simulink model "VSI_Space_Vector_PWM"  (R2020b)
settings: Solver=ode45  StartTime=0.0  StopTime=5/fc  MaxStep=1e-5  RelTol=1e-3  EnableMultiTasking=on
InitFcn:
  | Vdc=400;
  | Ts=2e-6; %Simulation sampling time
  | fc = 50;
  | fs = 10000;
  | shift = 0;
  | m = 1;
StopFcn:
  | clc
  | figure(1);
  | plot(a(:,1),a(:,2),'-b',b(:,1),b(:,2),'-r');
  | axis equal;
  | grid;
  | title('Space Vector PWM');
  | 
model workspace (MAT data in the model file):
  Param = Simulink.Parameter
  Param.Value = 25
  Param.DataType = 'auto'
  Param.Dimensions = [1 1]
  sw_array = reshape([0 0 0 1 0 0 1 1 0 1 1 1 1 1 0 1 0 0 0 0 0 0 0 0 0 1 0 1 1 0 1 1 1 1 1 0 0 1 0 0 0 0 0 0 0 0 1 0 0 1 1 1 1 1 0 1 1 0 1 0 0 0 0 0 0 0 0 0 1 0 1 1 1 1 1 0 1 1 0 0 1 0 0 0 0 0 0 0 0 1 1 0 1 1 1 1 1 0 1 0 0 1 0 0 0 0 0 0 1 0 0 1 0 1 1 1 1 1 0 1 1 0 0 0 0 0], [3 7 6])
libraries: powerlib x20, simulink x2
settings Model: Creator=sample  LastModifiedBy=Karim
settings DataIOCC: LimitDataPoints=on  SaveFormat=Array  SignalLoggingSaveFormat=ModelDataLogs  ReturnWorkspaceOutputs=off
settings OptimizationCC: ExpressionDepthLimit=2147483647  LifeSpan=inf
settings DebuggingCC: UnderspecifiedInitializationDetection=Classic  MergeDetectMultiDrivingBlocksExec=none  SolverPrmCheckMsg=warning  FcnCallInpInsideContextMsg=warning  StateNameClashWarn=warning  SFUnexpectedBacktrackingDiag=warning  SFNoUnconditionalDefaultTransitionDiag=warning  SFExecutionAtInitializationDiag=none  ArithmeticOperatorsInVariantConditions=warning
settings HardwareCC: ProdBitPerPointer=32  ProdBitPerSizeT=32  ProdBitPerPtrDiffT=32  ProdLargestAtomicFloat=None  ProdIntDivRoundTo=Undefined  ProdEndianess=Unspecified  ProdWordSize=32  ProdHWDeviceType=32-bit Generic
settings ModelReferenceCC: PropagateSignalLabelsOutOfModel=off
settings SFSimCC: SimUseLocalCustomCode=off  CustomCodeUndefinedFunction=UseInterfaceOnly
settings RTWCC: RTWUseLocalCustomCode=off
settings CodeAppCC: StateflowObjectComments=on
settings GRTTargetCC: TargetLangStandard=C89/C90 (ANSI)  CombineOutputUpdateFcns=off  GRTInterface=on
settings ConfigComp: CovMetricSettings=dw  CovSaveCumulativeToWorkspaceVar=on  CovSaveSingleToWorkspaceVar=on  CovExternalEMLEnable=off
settings SimscapeCC: SimscapeNormalizeSystem=off

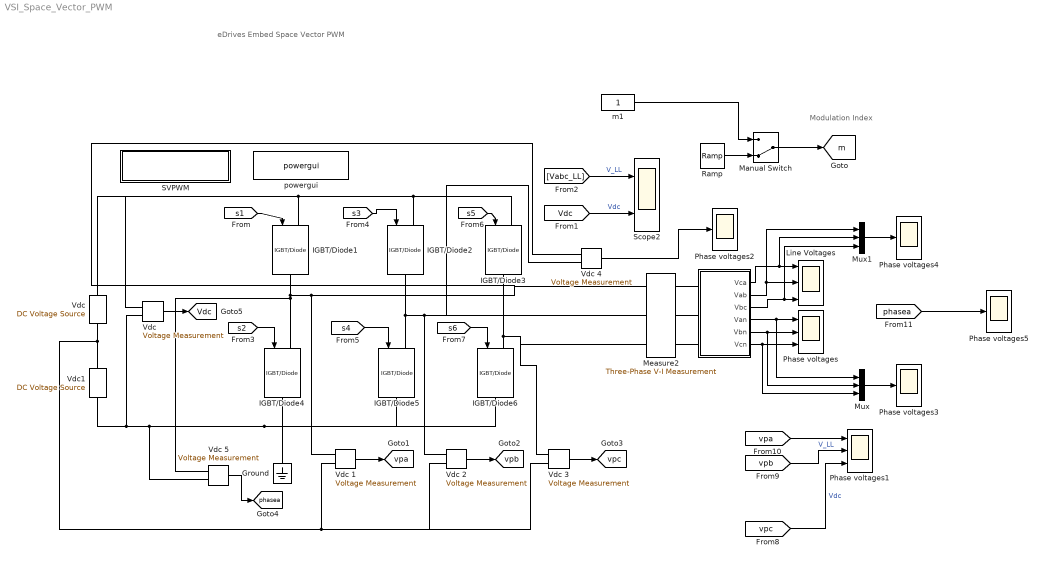
== system VSI_Space_Vector_PWM ==
  note: Modulation Index
  note: eDrives Embed
      |
      |   Space Vector  PWM
  " " : Subsystem
  Ground : powerlib/Elements/Ground  LConnTagsString=a
  IGBT/Diode{1..6} (6 alike) : powerlib/Power Electronics/IGBT//Diode  Ron=1e-3  Rs=1e5  Cs=inf  Measurements=off
  Line Voltages : Scope  NumInputPorts=3
  Manual Switch : ManualSwitch  CurrentSetting=0
  Measure2 : powerlib/Measurements/Three-Phase V-I Measurement  VoltageMeasurement=phase-to-phase  SetLabelV=on  LabelV=Vabc_LL  Vpu=off  VpuLL=off  CurrentMeasurement=no  SetLabelI=off  LabelI=I1  Ipu=off  Pbase=1e3  Vbase=380  OutputType=Magnitude  PhasorSimulation=off  PSBequivalent=0
  Mux : Mux  Inputs=3
  Mux1 : Mux  Inputs=3
  Phase voltages : Scope  NumInputPorts=3
  Phase voltages1 : Scope  NumInputPorts=3
  Phase voltages{2..5} (4 alike) : Scope
  Ramp : simulink/Sources/Ramp  slope=5  start=0  InitialOutput=0.5
  SVPWM : Subsystem
  Scope2 : Scope  NumInputPorts=2
  Vdc : powerlib/Electrical Sources/DC Voltage Source  Amplitude=200  Measurements=None
  Vdc {,1..5} (6 alike) : powerlib/Measurements/Voltage Measurement  Tag=PoWeRsYsTeMmEaSuReMeNt  PhasorSimulation=off  OutputType=Magnitude  PSBequivalent=0
  Vdc1 : powerlib/Electrical Sources/DC Voltage Source  Amplitude=200  Measurements=None
  m1 : Constant  SampleTime=Ts
  powergui : powerlib/powergui  Priority=1  SimulationMode=Discrete  SampleTime=1e-6  frequency=60  Iterations=50  frequencyindice=0  Pbase=100e6  ErrMax=1e-4  UnitsV=kV  UnitsW=MW  buscounter=0  FunctionMessages=off  echomessages=off  EnableUseOfTLC=off  CurrentSourceSwitches=off  DisableSnubberDevices=off  DisableRonSwitches=off  DisableVfSwitches=off  DisplayEquations=off  AutomaticDiscreteSolvers=off  SolverType=Tustin  Interpol=off  ExternalGateDelay=off  methode=off  Ts=0  x0status=blocks  SPID=on  SwTol=0  HookPort=off  NonlinearTolerance=1e-4  nMaxIteration=100  ContinueOnMaxIteration=off  RestoreLinks=warning  ResistiveCurrentMeasurement=off  Frange=[0:2:500]  Ylog=off  Xlog=on  ShowGrid=off  save=off  variable=ZData  structure=sv2  ZoomFFT=off  StartTime=0  cycles=2  DisplayStyle=1  fundamental=50  FreqAxis=on  MaxFrequency=650  frequencyindicesteady=1  RmsSteady=1  display=off
  tag scope: Vdc=global, m=global, phasea=global, vpa=global, vpb=global, vpc=global
  wires:
  "Vdc "/1 -> [Vdc]
  " "/4(Van) -> Mux/1, Phase voltages/1
  " "/5(Vbn) -> Mux/2, Phase voltages/2
  " "/6(Vcn) -> Mux/3, Phase voltages/3
  [Vabc_LL] -> Scope2/1  "V_LL"
  [Vdc] -> Scope2/2  "Vdc"
  [s1] -> IGBT/Diode1/1
  [s2] -> IGBT/Diode4/1
  [s3] -> IGBT/Diode2/1
  [s4] -> IGBT/Diode5/1
  [s5] -> IGBT/Diode3/1
  [s6] -> IGBT/Diode6/1
  " "/1(Vca) -> Mux1/2, Line Voltages/1
  " "/2(Vab) -> Mux1/1, Line Voltages/2
  " "/3(Vbc) -> Line Voltages/3, Mux1/3
  m1/1 -> Manual Switch/1
  Manual Switch/1 -> [m]
  Ramp/1 -> Manual Switch/2
  Vdc 1/1 -> [vpa]
  Vdc 2/1 -> [vpb]
  Vdc 3/1 -> [vpc]
  [vpb] -> Phase voltages1/2  "V_LL"
  [vpc] -> Phase voltages1/3  "Vdc"
  [vpa] -> Phase voltages1/1
  Vdc 4/1 -> Phase voltages2/1
  Mux/1 -> Phase voltages3/1
  Mux1/1 -> Phase voltages4/1
  Vdc 5/1 -> [phasea]
  [phasea] -> Phase voltages5/1
  connections:
  Measure2/RConn1 -- " "/LConn1
  Measure2/RConn2 -- " "/LConn2
  " "/LConn3 -- Measure2/RConn3
  IGBT/Diode2/LConn1 -- IGBT/Diode3/LConn1 -- Vdc/RConn1 -- "Vdc "/LConn1 -- IGBT/Diode1/LConn1
  IGBT/Diode1/RConn1 -- Measure2/LConn1 -- Vdc 4/LConn1 -- Vdc 1/LConn1 -- IGBT/Diode4/LConn1 -- Vdc 5/LConn1
  IGBT/Diode5/RConn1 -- IGBT/Diode6/RConn1 -- Ground/LConn1 -- IGBT/Diode4/RConn1 -- Vdc 5/LConn2 -- Vdc1/LConn1 -- "Vdc "/LConn2
  IGBT/Diode3/RConn1 -- Measure2/LConn3 -- Vdc 3/LConn1 -- IGBT/Diode6/LConn1
  IGBT/Diode5/LConn1 -- Measure2/LConn2 -- Vdc 4/LConn2 -- Vdc 2/LConn1 -- IGBT/Diode2/RConn1
  Vdc 1/LConn2 -- Vdc/LConn1 -- Vdc1/RConn1 -- Vdc 3/LConn2 -- Vdc 2/LConn2

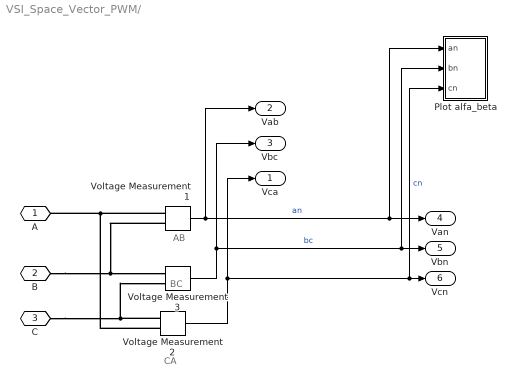
== system VSI_Space_Vector_PWM/  ==
  note: CA
  note: BC
  note: AB
  Plot alfa_beta : Subsystem
  Voltage Measurement1 : powerlib/Measurements/Voltage Measurement  PhasorSimulation=off  OutputType=Complex  PSBequivalent=0
  Voltage Measurement2 : powerlib/Measurements/Voltage Measurement  PhasorSimulation=off  OutputType=Complex  PSBequivalent=0
  Voltage Measurement3 : powerlib/Measurements/Voltage Measurement  PhasorSimulation=off  OutputType=Complex  PSBequivalent=0
  A : PMIOPort  Side=Left
  B : PMIOPort  Port=2  Side=Left
  C : PMIOPort  Port=3  Side=Left
  Vca : Outport
  Vab : Outport  Port=2
  Vbc : Outport  Port=3
  Van : Outport  Port=4
  Vbn : Outport  Port=5
  Vcn : Outport  Port=6
  wires:
  Voltage Measurement3/1 -> Plot alfa_beta/2(bn), Vbn/1, Vbc/1  "bc"
  Voltage Measurement1/1 -> Plot alfa_beta/1(an), Van/1, Vab/1  "an"
  Voltage Measurement2/1 -> Plot alfa_beta/3(cn), Vcn/1, Vca/1  "cn"
  connections:
  Voltage Measurement1/LConn2 -- B/RConn1 -- Voltage Measurement3/LConn1
  Voltage Measurement2/LConn1 -- C/RConn1 -- Voltage Measurement3/LConn2
  Voltage Measurement1/LConn1 -- Voltage Measurement2/LConn2 -- A/RConn1

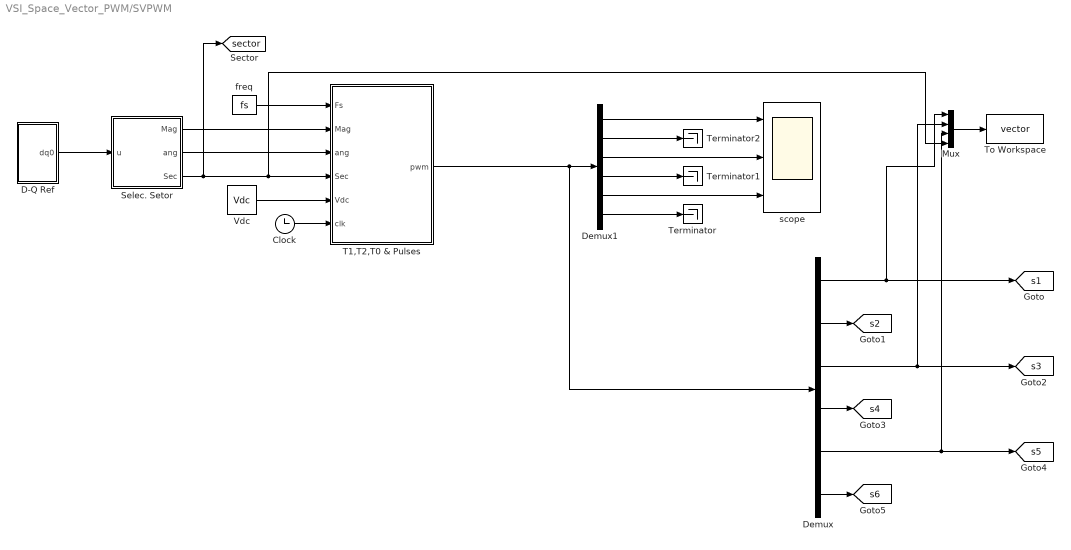
== system VSI_Space_Vector_PWM/SVPWM ==
  " T1,T2,T0 & Pulses" : MATLAB Function  TreatAsAtomicUnit=on
  " freq" : Constant  Value=fs
  Clock : Clock
      settings: Decimation=100
  "D-Q Ref " : Subsystem
  Demux : Demux  Outputs=6
  Demux1 : Demux  Outputs=6
  Mux : Mux
  Selec. Setor : MATLAB Function  TreatAsAtomicUnit=on
  Terminator : Terminator
  Terminator1 : Terminator
  Terminator2 : Terminator
  To Workspace : ToWorkspace  VariableName=vector  SampleTime=-1
  Vdc : Constant  Value=Vdc
  scope : Scope  NumInputPorts=3
  tag scope: s1=global, s2=global, s3=global, s4=global, s5=global, s6=global, sector=global
  wires:
  Selec. Setor/2(ang) -> " T1,T2,T0 & Pulses"/3(ang)
  Demux1/1 -> scope/1
  " freq"/1 -> " T1,T2,T0 & Pulses"/1(Fs)
  "D-Q Ref "/1(dq0) -> Selec. Setor/1(u)
  Selec. Setor/1(Mag) -> " T1,T2,T0 & Pulses"/2(Mag)
  Vdc/1 -> " T1,T2,T0 & Pulses"/5(Vdc)
  Selec. Setor/3(Sec) -> Mux/4, " T1,T2,T0 & Pulses"/4(Sec), [sector]
  Clock/1 -> " T1,T2,T0 & Pulses"/6(clk)
  Demux/1 -> Mux/1, [s1]
  Demux/2 -> [s2]
  Demux/3 -> Mux/2, [s3]
  Demux/4 -> [s4]
  Demux/6 -> [s6]
  " T1,T2,T0 & Pulses"/1(pwm) -> Demux/1, Demux1/1
  Demux1/3 -> scope/2
  Demux1/5 -> scope/3
  Demux1/6 -> Terminator/1
  Demux1/2 -> Terminator2/1
  Demux1/4 -> Terminator1/1
  Demux/5 -> Mux/3, [s5]
  Mux/1 -> To Workspace/1

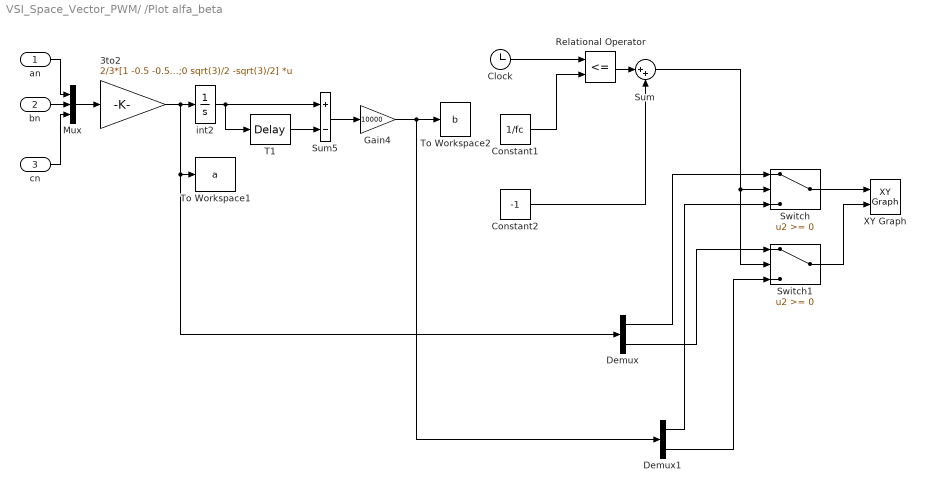
== system VSI_Space_Vector_PWM/ /Plot alfa_beta ==
  an : Inport
  bn : Inport  Port=2
  cn : Inport  Port=3
  3to2 : Gain  Gain=2/3*[1 -0.5 -0.5;0 sqrt(3)/2 -sqrt(3)/2]  Multiplication=Matrix(K*u)  SaturateOnIntegerOverflow=on  OutDataTypeStr=Inherit: Same as input  ParamDataTypeStr=Inherit: Same as input
  Clock : Clock
  Constant1 : Constant  Value=1/fc
  Constant2 : Constant  Value=-1
  Demux : Demux  Outputs=2
  Demux1 : Demux  Outputs=2
  Gain4 : Gain  Gain=10000  SaturateOnIntegerOverflow=on  OutDataTypeStr=Inherit: Same as input  ParamDataTypeStr=Inherit: Same as input
  Mux : Mux  Inputs=3
  Relational Operator : RelationalOperator  Operator=<=  OutDataTypeStr=boolean  RndMeth=Nearest
  Sum : Sum  Inputs=|++
  Sum5 : Sum  Inputs=+-  InputSameDT=on  SaturateOnIntegerOverflow=on  OutDataTypeStr=Inherit: Same as first input
  Switch : Switch
  Switch1 : Switch
  T1 : TransportDelay  DelayTime=1/10000  BufferSize=2048
  To Workspace1 : ToWorkspace  VariableName=a  SampleTime=-1
      settings: Decimation=2
  To Workspace2 : ToWorkspace  VariableName=b  SampleTime=-1
      settings: Decimation=2
  XY Graph : simulink/Sinks/XY Graph  xmin=-500  xmax=500  ymin=-500  ymax=500  st=-1
  int2 : Integrator
  wires:
  cn/1 -> Mux/3
  an/1 -> Mux/1
  Mux/1 -> 3to2/1
  bn/1 -> Mux/2
  Sum5/1 -> Gain4/1
  int2/1 -> Sum5/1, T1/1
  3to2/1 -> int2/1, Demux/1, To Workspace1/1
  T1/1 -> Sum5/2
  Gain4/1 -> Demux1/1, To Workspace2/1
  Relational Operator/1 -> Sum/1
  Demux/1 -> Switch/1
  Demux/2 -> Switch1/1
  Demux1/1 -> Switch/3
  Demux1/2 -> Switch1/3
  Clock/1 -> Relational Operator/1
  Constant1/1 -> Relational Operator/2
  Constant2/1 -> Sum/2
  Sum/1 -> Switch1/2, Switch/2
  Switch/1 -> XY Graph/1
  Switch1/1 -> XY Graph/2

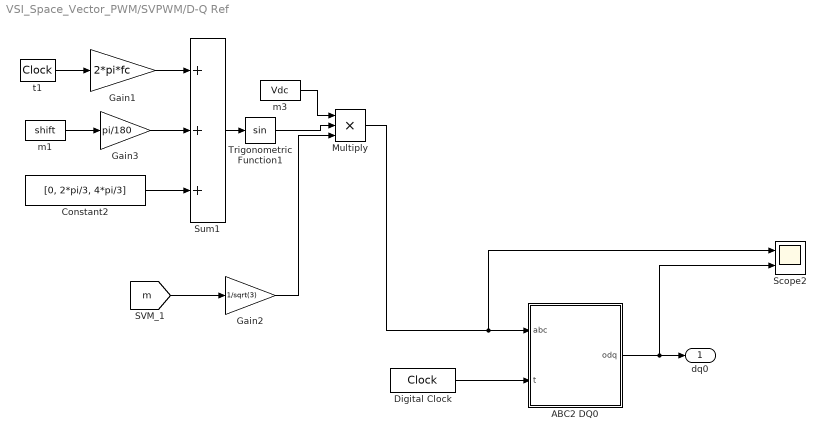
== system VSI_Space_Vector_PWM/SVPWM/D-Q Ref  ==
  ABC2 DQ0 : MATLAB Function  TreatAsAtomicUnit=on
  Constant2 : Constant  Value=[0, 2*pi/3, 4*pi/3]  SampleTime=-1
  Digital Clock : DigitalClock
  Gain1 : Gain  Gain=2*pi*fc  SaturateOnIntegerOverflow=on  OutDataTypeStr=Inherit: Same as input  ParamDataTypeStr=Inherit: Same as input
  Gain2 : Gain  Gain=1/sqrt(3)  SaturateOnIntegerOverflow=on  OutDataTypeStr=Inherit: Same as input  ParamDataTypeStr=Inherit: Same as input
  Gain3 : Gain  Gain=pi/180  SaturateOnIntegerOverflow=on  OutDataTypeStr=Inherit: Same as input  ParamDataTypeStr=Inherit: Same as input
  Multiply : Product  Inputs=***
  Scope2 : Scope  NumInputPorts=2
  Sum1 : Sum  Inputs=+++  InputSameDT=on  SaturateOnIntegerOverflow=on  OutDataTypeStr=Inherit: Same as first input
  Trigonometric Function1 : Trigonometry
  m1 : Constant  Value=shift  SampleTime=Ts
  m3 : Constant  Value=Vdc  SampleTime=2e-6
  t1 : DigitalClock  SampleTime=Ts
  dq0 : Outport
  wires:
  ABC2 DQ0/1(odq) -> Scope2/2, dq0/1
  Digital Clock/1 -> ABC2 DQ0/2(t)
  Sum1/1 -> Trigonometric Function1/1
  Constant2/1 -> Sum1/3
  m1/1 -> Gain3/1
  Gain3/1 -> Sum1/2
  Gain1/1 -> Sum1/1
  t1/1 -> Gain1/1
  m3/1 -> Multiply/1
  Trigonometric Function1/1 -> Multiply/2
  Gain2/1 -> Multiply/3
  Multiply/1 -> Scope2/1, ABC2 DQ0/1(abc)
  [m] -> Gain2/1

== matlab function VSI_Space_Vector_PWM/SVPWM/Selec. Setor ==
  data: Mag output; ang output; u input; Sec output
function [Mag,ang,Sec] = fcn(u)

complexo=u(2)+ i* u(3);
Mag=abs(complexo);
ang=atan2(imag(complexo),real(complexo));
alpha=ang*180/pi;

Sec = (alpha>0 & alpha<=60)*1+ (alpha>60 & alpha<=120)*2  + (alpha>120 & alpha<=180)*3 ...
  +(alpha>-180 & alpha<-120)*4+ (alpha>-120 & alpha<=-60)*5 + (alpha>-60 & alpha<=0)*6;

== matlab function VSI_Space_Vector_PWM/SVPWM/ T1,T2,T0 & Pulses ==
  data: Fs input; Mag input; ang input; Sec input; Vdc input; pwm output; clk input

% -----------------------------------------------------------------------    
%      eDrives Embed
%      Space Vector PWM

% ------------------------------------------------------------------------

% T1,T2,T0,timet
function pwm  = fcn(Fs,Mag,ang,Sec,Vdc,clk)

% Time synchronization with the simulink clock. 
t=clk;

% Vdc at workspace
% General expression for the calculation of T1, T2 and T0. 


T1=(sqrt(3)*(Mag/Vdc))*sin(Sec*pi/3 -ang)/Fs;
T2=(sqrt(3)*(Mag/Vdc))*sin(ang - ((Sec-1)*pi/3))/Fs;
T0= (1/Fs -T1- T2)/2;

% Change of sectors 
sec_ant=mod(floor(Sec),2);

if(sec_ant~=1)  % detection sector exchange
    
 T1=(sqrt(3)*(Mag/Vdc))*sin(ang - ((Sec-1)*pi/3))/Fs;
 T2=(sqrt(3)*(Mag/Vdc))*sin(Sec*pi/3 -ang)/Fs;
 
end


% Sawtooth
ref= 1/Fs * rem(t,1/Fs)/(1/Fs);


% Time intervals
int1=T0/4;
int2=int1+T1/2;
int3=int2+T2/2;
int4=int3+T0/2;
int5=int4+T2/2;
int6=int5+T1/2;

timet=1+(ref>=int1)+(ref>=int2)+(ref>=int3)+(ref>=int4)+(ref>=int5)+(ref>=int6);
% 
% 
sw_array=zeros(3,7,6);  %Initialize table of key states -> 3 rows (arms), 7 columns (times) and 6 vectors (sectors). 

%                ------Arm A --------   -------Arm B --------  -------Arm C --------
sw_array(:,:,1)=[0	1	1	1	1	1	0;0  0	1	1	1	0	0; 0	0	0	1	0	0	0]; %sector 1
sw_array(:,:,2)=[0	0	1	1	1	0	0;0	 1	1	1	1	1	0; 0	0	0	1	0	0	0]; %sector 2
sw_array(:,:,3)=[0	0	0	1	0	0	0;0	 1	1	1	1	1	0; 0	0	1	1	1	0	0]; %sector 3
sw_array(:,:,4)=[0	0	0	1	0	0	0;0	 0	1	1	1	0	0; 0	1	1	1	1	1	0]; %sector 4
sw_array(:,:,5)=[0	0	1	1	1	0	0;0	 0	0	1	0	0	0; 0	1	1	1	1	1	0]; %sector 5
sw_array(:,:,6)=[0	1	1	1	1	1	0;0	 0	0	1	0	0	0; 0	0	1	1	1	0	0]; %sector 6
 

if t<1e-6
Sec=1;
end;


    
S1=sw_array(1,timet,Sec);
S2= ~S1;
S3=sw_array(2,timet,Sec);
S4= ~S3;
S5=sw_array(3,timet,Sec);
S6= ~S5;
% SVPWM



pwm= [S1 S2 S3 S4 S5 S6];






end

== matlab function VSI_Space_Vector_PWM/SVPWM/D-Q Ref /ABC2 DQ0 ==
  data: abc input; odq output; t input
function odq = fcn(abc,t)

detla=2*pi*50*(t-5e-6) ; % f=50hz
a=abc(1);
b=abc(2);
c=abc(3);
T=[1/2          1/2                1/2;...
   cos(detla) cos(detla-2*pi/3)  cos(detla+2*pi/3);...
   sin(detla) sin(detla-2*pi/3)  sin(detla+2*pi/3)];

U=[a;b;c];


odq =2/3* T * U ;
